simulink model "sim1"  (Simulink 8.5)
settings: Solver=ode45  StartTime=0.0  StopTime=10.0  RelTol=1e-3
libraries: simulink x1
settings Model: Creator=alaa ahmed amer  LastModifiedBy=alaa ahmed amer
settings DataIOCC: SignalLoggingSaveFormat=Dataset
settings OptimizationCC: ExpressionDepthLimit=128
settings DebuggingCC: UnderspecifiedInitializationDetection=Simplified  MergeDetectMultiDrivingBlocksExec=error  FcnCallInpInsideContextMsg=EnableAllAsError  StateNameClashWarn=none
settings GRTTargetCC: CombineOutputUpdateFcns=on  GRTInterface=off

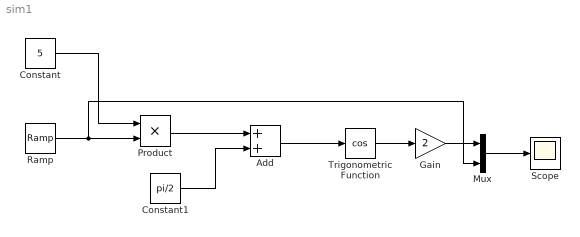
== system sim1 ==
  Add : Sum
  Constant : Constant  Value=5
  Constant1 : Constant  Value=pi/2
  Gain : Gain  Gain=2
  Mux : Mux  Inputs=2
  Product : Product
  Ramp : simulink/Sources/Ramp  slope=1  start=0  X0=0
  Scope : Scope
  Trigonometric Function : Trigonometry  Operator=cos
  wires:
  Ramp/1 -> Mux/2, Product/2
  Constant/1 -> Product/1
  Product/1 -> Add/1
  Constant1/1 -> Add/2
  Add/1 -> Trigonometric Function/1
  Trigonometric Function/1 -> Gain/1
  Mux/1 -> Scope/1
  Gain/1 -> Mux/1
